simulink model "Battery_Model_2nd_order(1)"  (R2014a)
settings: Solver=ode45  StartTime=0.0  StopTime=2000  RelTol=1e-3
values from neighbouring files (symbols this model uses):
  Em0 = 14.341    [Battery_estm.m]
  I_constant = 4    [Battery_estm.m]
  K = 0.11694    [Battery_estm.m]
  Rb = 0.007122    [Battery_estm.m]
  SOC_intial = 0.8    [Battery_estm.m]
settings Model: Creator=xp  LastModifiedBy=xp

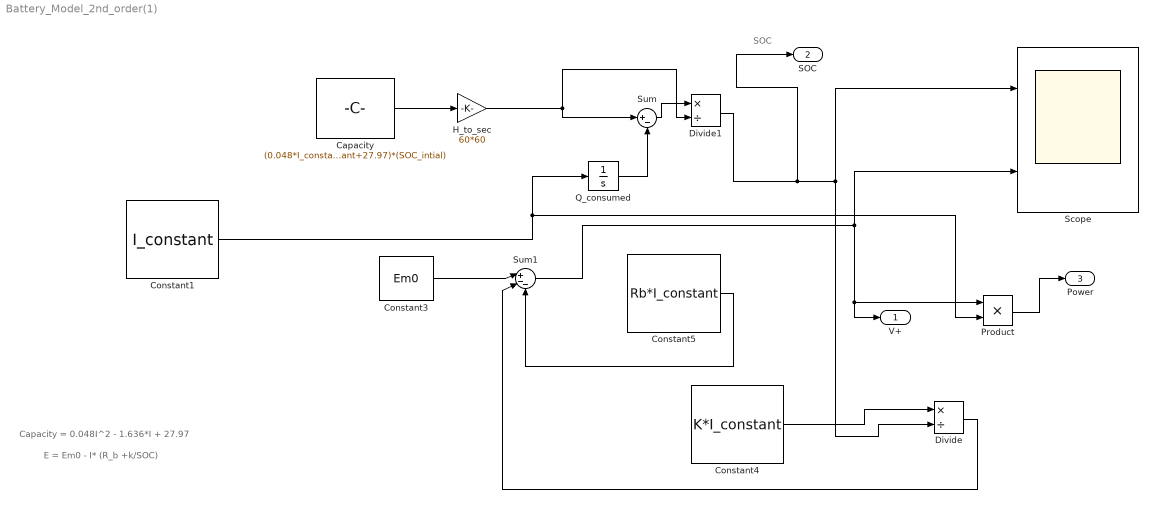
== system Battery_Model_2nd_order(1) ==
  note: Capacity = 0.048I^2 - 1.636*I + 27.97
  note: E = Em0 - I* (R_b +k/SOC)
  note: SOC
  Capacity : Constant  Value=(0.048*I_constant^2 -1.636*I_constant+27.97)*(SOC_intial)
  Constant1 : Constant  Value=I_constant
  Constant3 : Constant  Value=Em0
  Constant4 : Constant  Value=K*I_constant
  Constant5 : Constant  Value=Rb*I_constant
  Divide : Product  Inputs=*/
  Divide1 : Product  Inputs=*/
  H_to_sec : Gain  Gain=60*60
  Product : Product
  Q_consumed : Integrator
  Scope : Scope  NumInputPorts=2
      settings: YMin=-5~-5  YMax=5~5
  Sum : Sum  Inputs=|+-
  Sum1 : Sum  Inputs=|+--
  V+ : Outport
  SOC : Outport  Port=2
  Power : Outport  Port=3
  wires:
  Q_consumed/1 -> Sum/2
  Sum/1 -> Divide1/1
  Divide1/1 -> SOC/1, Divide/2, Scope/1
  Constant3/1 -> Sum1/1
  Sum1/1 -> Product/1, V+/1, Scope/2
  Constant4/1 -> Divide/1
  Divide/1 -> Sum1/2
  Constant5/1 -> Sum1/3
  Constant1/1 -> Q_consumed/1, Product/2
  Product/1 -> Power/1
  H_to_sec/1 -> Divide1/2, Sum/1
  Capacity/1 -> H_to_sec/1
